simulink model "Irradiancia"  (R2021a)
settings: Solver=VariableStepAuto  StartTime=0.0  StopTime=60  RelTol=1e-8
undefined symbols (not defined in the file or in its folder): sigbuilder_block
settings Model: Creator=Guillermo  LastModifiedBy=Guillermo
settings SolverCC: ZeroCrossAlgorithm=Adaptive

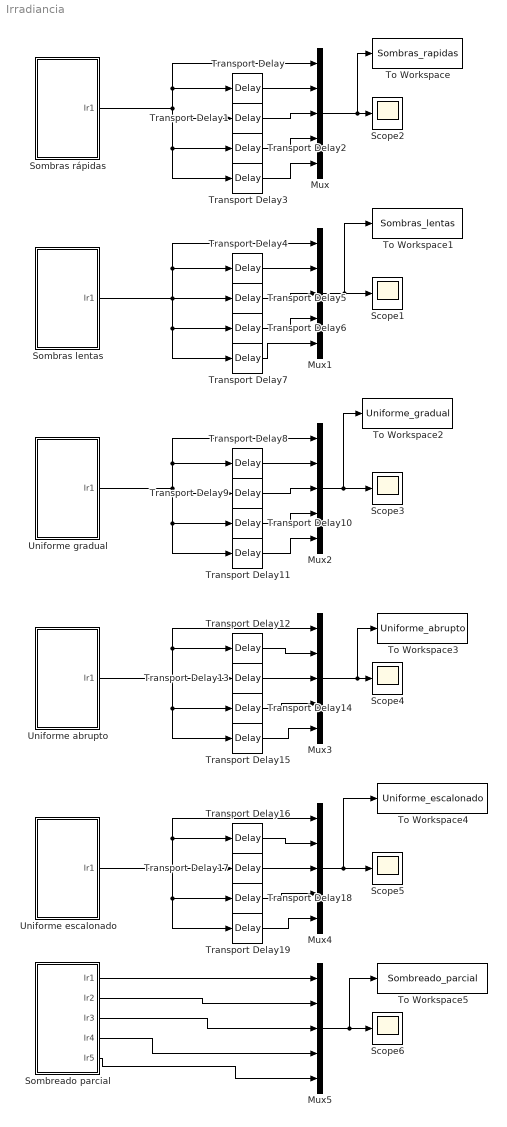
== system Irradiancia ==
  Mux{,1..5} (6 alike) : Mux  Inputs=5
  Scope{1..6} (6 alike) : Scope
  Sombras lentas : Subsystem  Tag=STV Subsys  LoadFcn=sigbuilder_block('load');  StartFcn=sigbuilder_block('start');  StopFcn=sigbuilder_block('stop');  ClipboardFcn=sigbuilder_block('clipboard');  mask(Sigbuilder block){tuvar=[0:10]}
      mask help: Simulink:masks:SigbuilderBlock_MD
      mask init:
      | if ~strcmp(get_param(bdroot(gcbh),'SimulationStatus'),'stopped') tuvar = sigbuilder_block('maskInit'); end
      settings: CopyFcn=sigbuilder_block('copy');  DeleteFcn=sigbuilder_block('delete');  ModelCloseFcn=sigbuilder_block('modelClose');  PreSaveFcn=sigbuilder_block('preSave');  PauseFcn=sigbuilder_block('pause');  ContinueFcn=sigbuilder_block('continue');  NameChangeFcn=sigbuilder_block('namechange');  OpenFcn=sigbuilder_block('open',[6 30 1908 951.75 ]);  CloseFcn=sigbuilder_block('close');
      mask Display: plot(0, 0, 100, 100,[2, 2, 32, 32, 2], [68, 8, 8, 68, 68],[32, 2], [38, 38], [32, 19, 2],[53, 60, 44], [32, 17, 17, 2],[16, 16, 31, 31]);txt = getActiveGroup(gcbh);text(2, 100, txt,'verticalAlignment', 'top');
  Sombras rápidas : Subsystem  Tag=STV Subsys  LoadFcn=sigbuilder_block('load');  StartFcn=sigbuilder_block('start');  StopFcn=sigbuilder_block('stop');  ClipboardFcn=sigbuilder_block('clipboard');  mask(Sigbuilder block){tuvar=[0:10]}
      mask help: Simulink:masks:SigbuilderBlock_MD
      mask init:
      | if ~strcmp(get_param(bdroot(gcbh),'SimulationStatus'),'stopped') tuvar = sigbuilder_block('maskInit'); end
      settings: CopyFcn=sigbuilder_block('copy');  DeleteFcn=sigbuilder_block('delete');  ModelCloseFcn=sigbuilder_block('modelClose');  PreSaveFcn=sigbuilder_block('preSave');  PauseFcn=sigbuilder_block('pause');  ContinueFcn=sigbuilder_block('continue');  NameChangeFcn=sigbuilder_block('namechange');  OpenFcn=sigbuilder_block('open',[59.25 144.75 1440 681.75 ]);  CloseFcn=sigbuilder_block('close');
      mask Display: plot(0, 0, 100, 100,[2, 2, 32, 32, 2], [68, 8, 8, 68, 68],[32, 2], [38, 38], [32, 19, 2],[53, 60, 44], [32, 17, 17, 2],[16, 16, 31, 31]);txt = getActiveGroup(gcbh);text(2, 100, txt,'verticalAlignment', 'top');
  Sombreado parcial : Subsystem  Tag=STV Subsys  LoadFcn=sigbuilder_block('load');  StartFcn=sigbuilder_block('start');  StopFcn=sigbuilder_block('stop');  ClipboardFcn=sigbuilder_block('clipboard');  mask(Sigbuilder block){tuvar=[0:10]}
      mask help: Simulink:masks:SigbuilderBlock_MD
      mask init:
      | if ~strcmp(get_param(bdroot(gcbh),'SimulationStatus'),'stopped') tuvar = sigbuilder_block('maskInit'); end
      settings: CopyFcn=sigbuilder_block('copy');  DeleteFcn=sigbuilder_block('delete');  ModelCloseFcn=sigbuilder_block('modelClose');  PreSaveFcn=sigbuilder_block('preSave');  PauseFcn=sigbuilder_block('pause');  ContinueFcn=sigbuilder_block('continue');  NameChangeFcn=sigbuilder_block('namechange');  OpenFcn=sigbuilder_block('open',[6 30 1908 951.75 ]);  CloseFcn=sigbuilder_block('close');
      mask Display: plot(0, 0, 100, 100,[2, 2, 32, 32, 2], [68, 8, 8, 68, 68],[32, 2], [38, 38], [32, 19, 2],[53, 60, 44], [32, 17, 17, 2],[16, 16, 31, 31]);txt = getActiveGroup(gcbh);text(2, 100, txt,'verticalAlignment', 'top');
  To Workspace : ToWorkspace  VariableName=Sombras_rapidas  SampleTime=1e-3
  To Workspace1 : ToWorkspace  VariableName=Sombras_lentas  SampleTime=1e-3
  To Workspace2 : ToWorkspace  VariableName=Uniforme_gradual  SampleTime=1e-3
  To Workspace3 : ToWorkspace  VariableName=Uniforme_abrupto  SampleTime=1e-3
  To Workspace4 : ToWorkspace  VariableName=Uniforme_escalonado  SampleTime=1e-3
  To Workspace5 : ToWorkspace  VariableName=Sombreado_parcial  SampleTime=1e-3
  Transport Delay : TransportDelay  DelayTime=0.1  InitialOutput=910
  Transport Delay1 : TransportDelay  DelayTime=0.2  InitialOutput=910
  Transport Delay10 : TransportDelay  DelayTime=0.3  InitialOutput=1000
  Transport Delay11 : TransportDelay  DelayTime=0.4  InitialOutput=1000
  Transport Delay12 : TransportDelay  DelayTime=0.1  InitialOutput=1000
  Transport Delay13 : TransportDelay  DelayTime=0.2  InitialOutput=1000
  Transport Delay14 : TransportDelay  DelayTime=0.3  InitialOutput=1000
  Transport Delay15 : TransportDelay  DelayTime=0.4  InitialOutput=1000
  Transport Delay16 : TransportDelay  DelayTime=0.1  InitialOutput=1000
  Transport Delay17 : TransportDelay  DelayTime=0.2  InitialOutput=1000
  Transport Delay18 : TransportDelay  DelayTime=0.3  InitialOutput=1000
  Transport Delay19 : TransportDelay  DelayTime=0.4  InitialOutput=1000
  Transport Delay2 : TransportDelay  DelayTime=0.3  InitialOutput=910
  Transport Delay3 : TransportDelay  DelayTime=0.4  InitialOutput=910
  Transport Delay4 : TransportDelay  DelayTime=0.1  InitialOutput=910
  Transport Delay5 : TransportDelay  DelayTime=0.2  InitialOutput=910
  Transport Delay6 : TransportDelay  DelayTime=0.3  InitialOutput=910
  Transport Delay7 : TransportDelay  DelayTime=0.4  InitialOutput=910
  Transport Delay8 : TransportDelay  DelayTime=0.1  InitialOutput=1000
  Transport Delay9 : TransportDelay  DelayTime=0.2  InitialOutput=1000
  Uniforme abrupto : Subsystem  Tag=STV Subsys  LoadFcn=sigbuilder_block('load');  StartFcn=sigbuilder_block('start');  StopFcn=sigbuilder_block('stop');  ClipboardFcn=sigbuilder_block('clipboard');  mask(Sigbuilder block){tuvar=[0:10]}
      mask help: Simulink:masks:SigbuilderBlock_MD
      mask init:
      | if ~strcmp(get_param(bdroot(gcbh),'SimulationStatus'),'stopped') tuvar = sigbuilder_block('maskInit'); end
      settings: CopyFcn=sigbuilder_block('copy');  DeleteFcn=sigbuilder_block('delete');  ModelCloseFcn=sigbuilder_block('modelClose');  PreSaveFcn=sigbuilder_block('preSave');  PauseFcn=sigbuilder_block('pause');  ContinueFcn=sigbuilder_block('continue');  NameChangeFcn=sigbuilder_block('namechange');  OpenFcn=sigbuilder_block('open',[6 30 1908 951.75 ]);  CloseFcn=sigbuilder_block('close');
      mask Display: plot(0, 0, 100, 100,[2, 2, 32, 32, 2], [68, 8, 8, 68, 68],[32, 2], [38, 38], [32, 19, 2],[53, 60, 44], [32, 17, 17, 2],[16, 16, 31, 31]);txt = getActiveGroup(gcbh);text(2, 100, txt,'verticalAlignment', 'top');
  Uniforme escalonado : Subsystem  Tag=STV Subsys  LoadFcn=sigbuilder_block('load');  StartFcn=sigbuilder_block('start');  StopFcn=sigbuilder_block('stop');  ClipboardFcn=sigbuilder_block('clipboard');  mask(Sigbuilder block){tuvar=[0:10]}
      mask help: Simulink:masks:SigbuilderBlock_MD
      mask init:
      | if ~strcmp(get_param(bdroot(gcbh),'SimulationStatus'),'stopped') tuvar = sigbuilder_block('maskInit'); end
      settings: CopyFcn=sigbuilder_block('copy');  DeleteFcn=sigbuilder_block('delete');  ModelCloseFcn=sigbuilder_block('modelClose');  PreSaveFcn=sigbuilder_block('preSave');  PauseFcn=sigbuilder_block('pause');  ContinueFcn=sigbuilder_block('continue');  NameChangeFcn=sigbuilder_block('namechange');  OpenFcn=sigbuilder_block('open',[6 30 1908 951.75 ]);  CloseFcn=sigbuilder_block('close');
      mask Display: plot(0, 0, 100, 100,[2, 2, 32, 32, 2], [68, 8, 8, 68, 68],[32, 2], [38, 38], [32, 19, 2],[53, 60, 44], [32, 17, 17, 2],[16, 16, 31, 31]);txt = getActiveGroup(gcbh);text(2, 100, txt,'verticalAlignment', 'top');
  Uniforme gradual : Subsystem  Tag=STV Subsys  LoadFcn=sigbuilder_block('load');  StartFcn=sigbuilder_block('start');  StopFcn=sigbuilder_block('stop');  ClipboardFcn=sigbuilder_block('clipboard');  mask(Sigbuilder block){tuvar=[0:10]}
      mask help: Simulink:masks:SigbuilderBlock_MD
      mask init:
      | if ~strcmp(get_param(bdroot(gcbh),'SimulationStatus'),'stopped') tuvar = sigbuilder_block('maskInit'); end
      settings: CopyFcn=sigbuilder_block('copy');  DeleteFcn=sigbuilder_block('delete');  ModelCloseFcn=sigbuilder_block('modelClose');  PreSaveFcn=sigbuilder_block('preSave');  PauseFcn=sigbuilder_block('pause');  ContinueFcn=sigbuilder_block('continue');  NameChangeFcn=sigbuilder_block('namechange');  OpenFcn=sigbuilder_block('open',[6 30 1908 951.75 ]);  CloseFcn=sigbuilder_block('close');
      mask Display: plot(0, 0, 100, 100,[2, 2, 32, 32, 2], [68, 8, 8, 68, 68],[32, 2], [38, 38], [32, 19, 2],[53, 60, 44], [32, 17, 17, 2],[16, 16, 31, 31]);txt = getActiveGroup(gcbh);text(2, 100, txt,'verticalAlignment', 'top');
  wires:
  Mux/1 -> To Workspace/1, Scope2/1
  Sombras rápidas/1(Ir1) -> Transport Delay3/1, Transport Delay2/1, Transport Delay1/1, Mux/1, Transport Delay/1
  Transport Delay/1 -> Mux/2
  Transport Delay1/1 -> Mux/3
  Transport Delay2/1 -> Mux/4
  Transport Delay3/1 -> Mux/5
  Transport Delay5/1 -> Mux1/3
  Transport Delay4/1 -> Mux1/2
  Transport Delay6/1 -> Mux1/4
  Transport Delay7/1 -> Mux1/5
  Sombras lentas/1(Ir1) -> Mux1/1, Transport Delay4/1, Transport Delay7/1, Transport Delay6/1, Transport Delay5/1
  Mux1/1 -> To Workspace1/1, Scope1/1
  Transport Delay9/1 -> Mux2/3
  Transport Delay8/1 -> Mux2/2
  Transport Delay10/1 -> Mux2/4
  Transport Delay11/1 -> Mux2/5
  Uniforme gradual/1(Ir1) -> Mux2/1, Transport Delay8/1, Transport Delay11/1, Transport Delay10/1, Transport Delay9/1
  Mux2/1 -> To Workspace2/1, Scope3/1
  Transport Delay13/1 -> Mux3/3
  Transport Delay12/1 -> Mux3/2
  Transport Delay14/1 -> Mux3/4
  Transport Delay15/1 -> Mux3/5
  Uniforme abrupto/1(Ir1) -> Mux3/1, Transport Delay12/1, Transport Delay13/1, Transport Delay15/1, Transport Delay14/1
  Mux3/1 -> To Workspace3/1, Scope4/1
  Uniforme escalonado/1(Ir1) -> Mux4/1, Transport Delay16/1, Transport Delay17/1, Transport Delay19/1, Transport Delay18/1
  Mux4/1 -> To Workspace4/1, Scope5/1
  Transport Delay19/1 -> Mux4/5
  Transport Delay18/1 -> Mux4/4
  Transport Delay17/1 -> Mux4/3
  Transport Delay16/1 -> Mux4/2
  Mux5/1 -> To Workspace5/1, Scope6/1
  Sombreado parcial/1(Ir1) -> Mux5/1
  Sombreado parcial/2(Ir2) -> Mux5/2
  Sombreado parcial/3(Ir3) -> Mux5/3
  Sombreado parcial/4(Ir4) -> Mux5/4
  Sombreado parcial/5(Ir5) -> Mux5/5

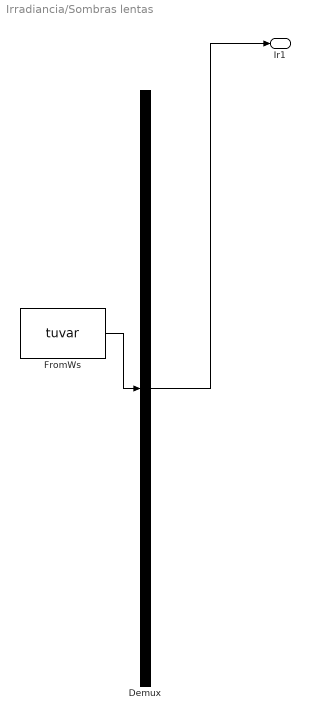
== system Irradiancia/Sombras lentas ==
  Demux : Demux  Tag=STV Demux  Outputs=1
      settings: DisplayOption=none
  FromWs : FromWorkspace  Tag=STV FromWs  VariableName=tuvar
      SigBuilderData=|
      | common.afterFinalStr = 'Extrapolate'
      | common.sampleTime = 0
      | dataSet.timeRange = [0 60]
      | dataSet.name = 'Group 1'
      | sbobj.Groups.Name = 'Group 1'
      | sbobj.Groups.Signals.Name = 'Ir1'
      | sbobj.Groups.Signals.XData = [0 1 1.4 7 7.25 16.5 16.75 25.25 25.75 34.75 35 37 37.25 45 45.25 48 48.25 50 50.25 57 57.25 60]
      | sbobj.Groups.Signals.YData = [910 500 295 295 910 910 295 295 910 910 295 295 910 910 295 295 910 910 295 295 910 910]
      | sbobj.Groups.TimeRange = [0 60]
  Ir1 : Outport  Tag=STV Outport
  wires:
  FromWs/1 -> Demux/1
  Demux/1 -> Ir1/1

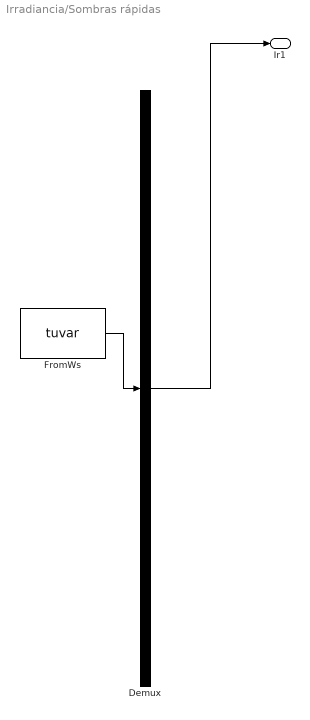
== system Irradiancia/Sombras rápidas ==
  Demux : Demux  Tag=STV Demux  Outputs=1
      settings: DisplayOption=none
  FromWs : FromWorkspace  Tag=STV FromWs  VariableName=tuvar
      SigBuilderData=|
      | common.afterFinalStr = 'Extrapolate'
      | common.sampleTime = 0
      | dataSet.timeRange = [0 60]
      | dataSet.name = 'Group 1'
      | sbobj.Groups.Name = 'Group 1'
      | sbobj.Groups.Signals.Name = 'Ir1'
      | sbobj.Groups.Signals.XData = [0 1 1.4 7 7.25 10 10.25 10.5 12 12.25 16 16.25 16.5 16.75 18.95 19.5 20 21.05 24 24.5 25 25.25 25.75 29 32 32.25 34 34.25 34.5 34.75 35 37 37.25 41 41.25 41.5 41.75 42 45 45.25 48 48.25 50 50.25 53.75 54 54.25 57 57.25 60]
      | sbobj.Groups.Signals.YData = [910 500 295 295 910 910 295 295 295 910 910 295 910 295 295 910 295 910 910 290 910 295 910 910 910 295 295 910 295 910 295 295 910 910 295 910 295 910 910 295 295 910 910 295 295 910 295 295 910 910]
      | sbobj.Groups.TimeRange = [0 60]
  Ir1 : Outport  Tag=STV Outport
  wires:
  FromWs/1 -> Demux/1
  Demux/1 -> Ir1/1

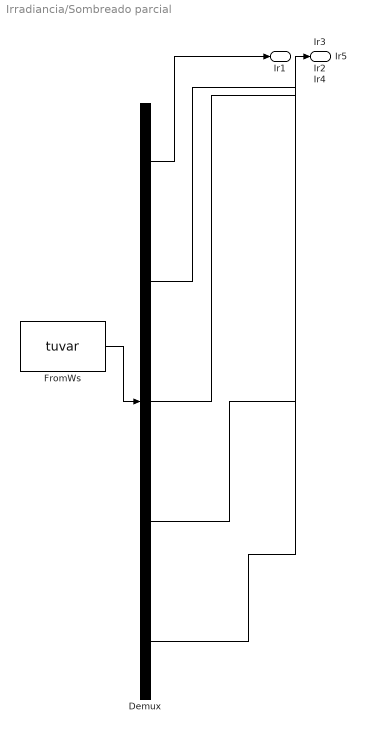
== system Irradiancia/Sombreado parcial ==
  Demux : Demux  Tag=STV Demux  Outputs=5
      settings: DisplayOption=none
  FromWs : FromWorkspace  Tag=STV FromWs  VariableName=tuvar
      SigBuilderData=|
      | common.afterFinalStr = 'Extrapolate'
      | common.sampleTime = 0
      | dataSet.timeRange = [0 60]
      | dataSet.name = 'Group 1'
      | sbobj.Groups.Name = 'Group 1'
      | sbobj.Groups.Signals(1).Name = 'Ir1'
      | sbobj.Groups.Signals(1).XData = [0 30 30.25 60]
      | sbobj.Groups.Signals(1).YData = [900 900 300 300]
      | sbobj.Groups.Signals(2).Name = 'Ir2'
      | sbobj.Groups.Signals(2).XData = [0 30 30.25 60]
      | sbobj.Groups.Signals(2).YData = [900 900 300 300]
      | sbobj.Groups.Signals(3).Name = 'Ir3'
      | sbobj.Groups.Signals(3).XData = [0 30 30.25 60]
      | sbobj.Groups.Signals(3).YData = [900 900 300 300]
      | sbobj.Groups.Signals(4).Name = 'Ir4'
      | sbobj.Groups.Signals(4).XData = [0 30 30.25 60]
      | sbobj.Groups.Signals(4).YData = [300 300 900 900]
      | sbobj.Groups.Signals(5).Name = 'Ir5'
      | sbobj.Groups.Signals(5).XData = [0 30 30.25 60]
      | sbobj.Groups.Signals(5).YData = [300 300 900 900]
      | sbobj.Groups.TimeRange = [0 60]
  Ir1 : Outport  Tag=STV Outport
  Ir2 : Outport  Tag=STV Outport  Port=2
  Ir3 : Outport  Tag=STV Outport  Port=3
  Ir4 : Outport  Tag=STV Outport  Port=4
  Ir5 : Outport  Tag=STV Outport  Port=5
  wires:
  FromWs/1 -> Demux/1
  Demux/1 -> Ir1/1
  Demux/2 -> Ir2/1
  Demux/3 -> Ir3/1
  Demux/4 -> Ir4/1
  Demux/5 -> Ir5/1

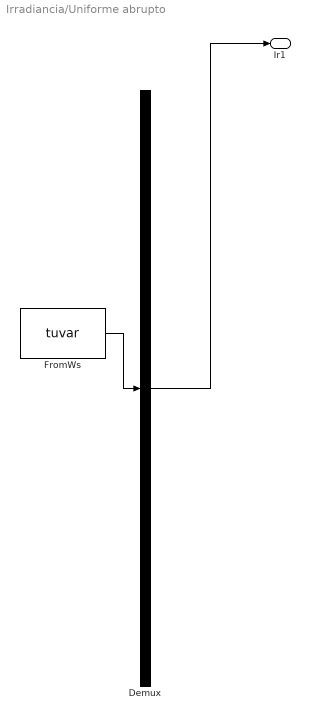
== system Irradiancia/Uniforme abrupto ==
  Demux : Demux  Tag=STV Demux  Outputs=1
      settings: DisplayOption=none
  FromWs : FromWorkspace  Tag=STV FromWs  VariableName=tuvar
      SigBuilderData=|
      | common.afterFinalStr = 'Extrapolate'
      | common.sampleTime = 0
      | dataSet.timeRange = [0 60]
      | dataSet.name = 'Group 1'
      | sbobj.Groups.Name = 'Group 1'
      | sbobj.Groups.Signals.Name = 'Ir1'
      | sbobj.Groups.Signals.XData = [0 30 30.25 60]
      | sbobj.Groups.Signals.YData = [1000 1000 200 200]
      | sbobj.Groups.TimeRange = [0 60]
  Ir1 : Outport  Tag=STV Outport
  wires:
  FromWs/1 -> Demux/1
  Demux/1 -> Ir1/1

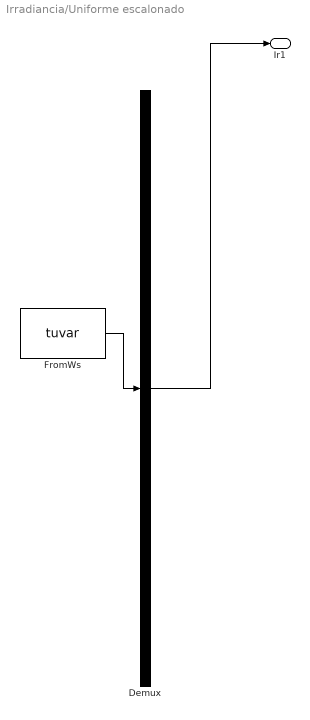
== system Irradiancia/Uniforme escalonado ==
  Demux : Demux  Tag=STV Demux  Outputs=1
      settings: DisplayOption=none
  FromWs : FromWorkspace  Tag=STV FromWs  VariableName=tuvar
      SigBuilderData=|
      | common.afterFinalStr = 'Extrapolate'
      | common.sampleTime = 0
      | dataSet.timeRange = [0 60]
      | dataSet.name = 'Group 1'
      | sbobj.Groups.Name = 'Group 1'
      | sbobj.Groups.Signals.Name = 'Ir1'
      | sbobj.Groups.Signals.XData = [0 15 15.25 30 30.25 45 45.25 60]
      | sbobj.Groups.Signals.YData = [1000 1000 800 800 600 600 400 400]
      | sbobj.Groups.TimeRange = [0 60]
  Ir1 : Outport  Tag=STV Outport
  wires:
  FromWs/1 -> Demux/1
  Demux/1 -> Ir1/1

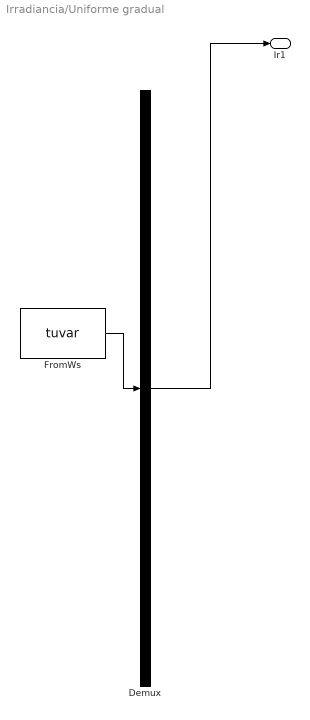
== system Irradiancia/Uniforme gradual ==
  Demux : Demux  Tag=STV Demux  Outputs=1
      settings: DisplayOption=none
  FromWs : FromWorkspace  Tag=STV FromWs  VariableName=tuvar
      SigBuilderData=|
      | common.afterFinalStr = 'Extrapolate'
      | common.sampleTime = 0
      | dataSet.timeRange = [0 60]
      | dataSet.name = 'Group 1'
      | sbobj.Groups.Name = 'Group 1'
      | sbobj.Groups.Signals.Name = 'Ir1'
      | sbobj.Groups.Signals.XData = [0 60]
      | sbobj.Groups.Signals.YData = [1000 200]
      | sbobj.Groups.TimeRange = [0 60]
  Ir1 : Outport  Tag=STV Outport
  wires:
  FromWs/1 -> Demux/1
  Demux/1 -> Ir1/1
